simulink model "Test_N5"  (R2020b)
settings: Solver=ode3  StartTime=0.0  StopTime=inf  FixedStep=0.05  RelTol=1e-3
libraries: XBotBlockToolbox x3, simulink x1, Utilities x1

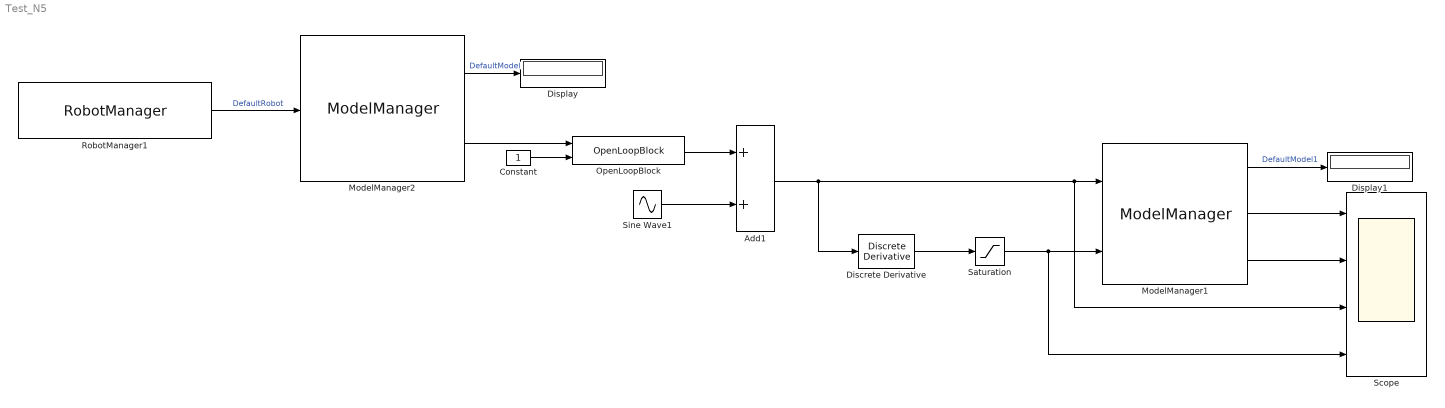
== system Test_N5 ==
  Add1 : Sum
  Constant : Constant
  Discrete Derivative : simulink/Discrete/Discrete Derivative  gainval=1.0  ICPrevScaledInput=0.0  OutMin=[]  OutMax=[]  OutDataType=fixdt(1, 16)  OutScaling=2^-10  DoSatur=off
  Display : Display
  Display1 : Display
  ModelManager1 : XBotBlockToolbox/ModelManager  ModelName=DefaultModel1  RobotName=DefaultRobot  UseExtModel=Off  SyncWithRobot=Off  GetFloatingBaseList={}  SetFloatingBaseComponent=Off  GravityRequest=Off  ReadingsList={ 'qM', 'qMdot' }  MechanicalLimitsList={}  ReferencesList={ 'qM_ref', 'qMdot_ref' }  OldModelName=DefaultModel1
  ModelManager2 : XBotBlockToolbox/ModelManager  ModelName=DefaultModel  RobotName=DefaultRobot  UseExtModel=Off  SyncWithRobot=On  GetFloatingBaseList={}  SetFloatingBaseComponent=Off  GravityRequest=Off  ReadingsList={ 'qM' }  MechanicalLimitsList={}  ReferencesList={}  OldModelName=DefaultModel
  OpenLoopBlock : Utilities/OpenLoopBlock  SystemSampleTime=-1  VariantActivationTime=update diagram  Latency=0  AutoFrameSizeCalculation=off
  RobotManager1 : XBotBlockToolbox/RobotManager  RobotName=DefaultRobot  ModelName=DefaultModel  UseExtRobot=Off  SyncWithModel=Off  ReadingsList={}  MechanicalLimitsList={}  ReferencesList={}  OldRobotName=DefaultRobot
  Saturation : Saturate  UpperLimit=1  LowerLimit=-1
  Scope : Scope  NumInputPorts=4
  Sine Wave1 : Sin  SampleTime=0
  wires:
  Add1/1 -> Scope/3, ModelManager1/1, Discrete Derivative/1
  Discrete Derivative/1 -> Saturation/1
  Sine Wave1/1 -> Add1/2
  Saturation/1 -> Scope/4, ModelManager1/2
  OpenLoopBlock/1 -> Add1/1
  ModelManager2/2 -> OpenLoopBlock/1
  RobotManager1/1 -> ModelManager2/1  "DefaultRobot"
  ModelManager2/1 -> Display/1  "DefaultModel"
  ModelManager1/1 -> Display1/1  "DefaultModel1"
  ModelManager1/2 -> Scope/1
  ModelManager1/3 -> Scope/2
  Constant/1 -> OpenLoopBlock/2
